simulink model "q_torsion"  (R2024a)
settings: Solver=ode1  StartTime=0.0  StopTime=5  FixedStep=0.002  RelTol=1e-3  EnableMultiTasking=on
values from neighbouring files (symbols this model uses):
  K = db2mag(12.15)    [pid_design.m]    (also in setup_torsion.m = d_torsion_1d_lqr(A,B))
  K_AMP = 1    [setup_torsion.m]
  K_ENC = 0    [config_srv02.m]
  VMAX_AMP = 0    [config_srv02.m]
  VMAX_DAC = 10    [setup_torsion.m]
  wcf = 2 * pi * 50.0    (= 314.159265359)    [setup_torsion.m]
  zetaf = 0.9    [setup_torsion.m]
undefined symbols (not defined in the file or in its folder): HIL, qc_get_step_size
libraries: quarc_library x9, simulink_extras x3
settings Model: SimulationMode=external  ExtModeTrigDuration=10000  Creator=MLevis  LastModifiedBy=quarc_user
settings SolverCC: AlgebraicLoopSolver=TrustRegion  PositivePriorityOrder=on
settings DataIOCC: LimitDataPoints=on  SaveFormat=Array  SignalLoggingSaveFormat=ModelDataLogs  ReturnWorkspaceOutputs=off
settings OptimizationCC: ExpressionDepthLimit=2147483647  InitFltsAndDblsToZero=on
settings DebuggingCC: SaveWithParameterizedLinksMsg=none  UnderspecifiedInitializationDetection=Classic  MergeDetectMultiDrivingBlocksExec=none  SolverPrmCheckMsg=warning  FcnCallInpInsideContextMsg=warning  UnconnectedInputMsg=warning  UnconnectedOutputMsg=warning  UnconnectedLineMsg=warning  StateNameClashWarn=warning  SFUnexpectedBacktrackingDiag=warning  SFNoUnconditionalDefaultTransitionDiag=warning  SFExecutionAtInitializationDiag=none  ArithmeticOperatorsInVariantConditions=warning
settings ModelReferenceCC: PropagateSignalLabelsOutOfModel=off
settings SFSimCC: SimUseLocalCustomCode=off  CustomCodeUndefinedFunction=UseInterfaceOnly
settings RTWCC: Description=QUARC Win64 Target Using Toolchain  SystemTargetFile=quarc_win64.tlc  TemplateMakefile=quarc_default_tmf  RTWUseLocalCustomCode=off  Toolchain=QUARC win64 | nmake (64-bit Windows)  BuildConfiguration=Faster Runs  GPUComputeCapability=3.5
settings CodeAppCC: StateflowObjectComments=on
settings STFCustomTargetCC: TargetLangStandard=C89/C90 (ANSI)  ConcurrentExecutionCompliant=on  SystemTargetFile=quarc_win64.tlc
settings GRTTargetCC: TargetLangStandard=C89/C90 (ANSI)  ParMdlRefBuildCompliant=off  CompOptLevelCompliant=off  CombineOutputUpdateFcns=off  MatFileLogging=off  CPPClassGenCompliant=off  GRTInterface=on  ExtMode=on  ExtModeMexFile=quarc_comm
settings ConfigComp: CovMetricSettings=dw  CovSaveCumulativeToWorkspaceVar=on  CovSaveSingleToWorkspaceVar=on  CovExternalEMLEnable=off

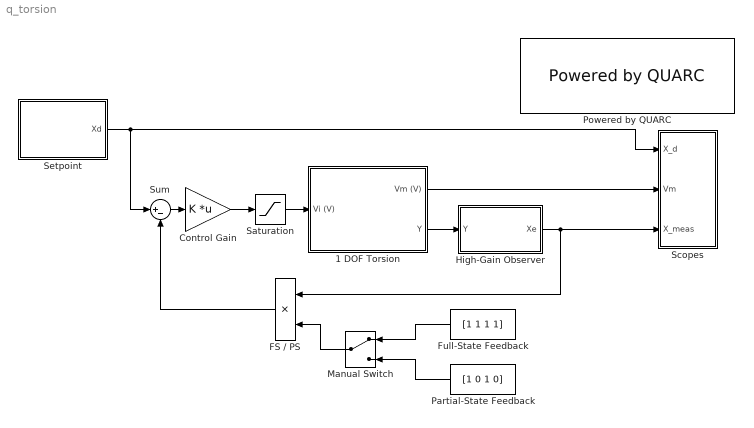
== system q_torsion ==
  1 DOF Torsion : Subsystem
  Control Gain : Gain  Gain=K  Multiplication=Matrix(K*u)  SaturateOnIntegerOverflow=on  OutDataTypeStr=Inherit: Same as input  ParamDataTypeStr=Inherit: Same as input
  FS / PS : Product  RndMeth=Zero
  Full-State Feedback : Constant  Value=[1 1 1 1]
  High-Gain Observer : Subsystem
  Manual Switch : ManualSwitch
  Partial-State Feedback : Constant  Value=[1 0 1 0]
  Powered by QUARC : quarc_library/Logos/Powered by QUARC
  Saturation : Saturate  UpperLimit=10  LowerLimit=-10
  Scopes : Subsystem
  Setpoint : Subsystem
  Sum : Sum  Inputs=|+-
  wires:
  1 DOF Torsion/2(Y) -> High-Gain Observer/1(Y)
  High-Gain Observer/1(Xe) -> Scopes/3(X_meas), FS / PS/1
  1 DOF Torsion/1(Vm (V)) -> Scopes/2(Vm)
  Setpoint/1(Xd) -> Scopes/1(X_d), Sum/1
  Full-State Feedback/1 -> Manual Switch/1
  Partial-State Feedback/1 -> Manual Switch/2
  Control Gain/1 -> Saturation/1
  Manual Switch/1 -> FS / PS/2
  FS / PS/1 -> Sum/2
  Sum/1 -> Control Gain/1
  Saturation/1 -> 1 DOF Torsion/1(Vi (V))

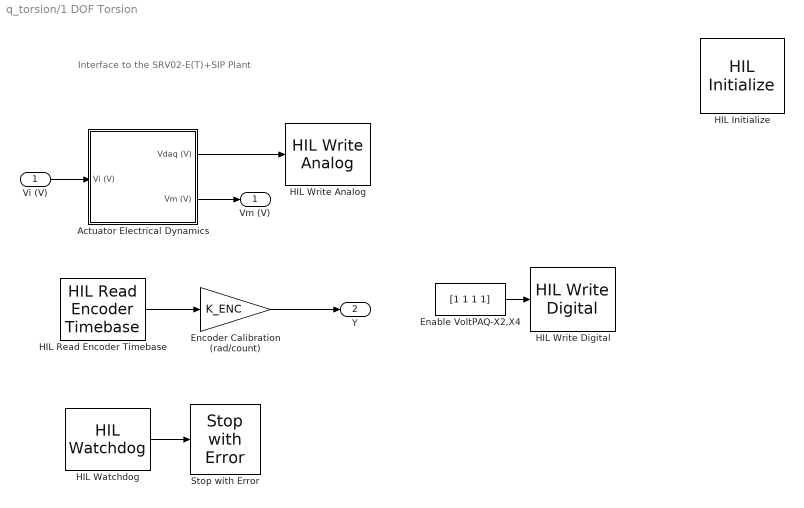
== system q_torsion/1 DOF Torsion ==
  note: Interface to the SRV02-E(T)+SIP Plant
  Vi (V) : Inport
  Actuator Electrical Dynamics : Subsystem
  Enable VoltPAQ-X2,X4 : Constant  Value=[1 1 1 1]
  Encoder Calibration (rad/count) : Gain  Gain=K_ENC  SaturateOnIntegerOverflow=on  OutDataTypeStr=Inherit: Same as input  ParamDataTypeStr=Inherit: Same as input
  HIL Initialize : quarc_library/Data Acquisition/Generic/Configuration/HIL Initialize  object_name=HIL-1  board_type=q2_usb  board_number=0  board_options=d0=digital;d1=digital;led=auto;update_rate=normal  exclusive=off  active=off  hardware_clocks=[0:2]  clock_modes=[]  initial_clock_frequencies=[]  set_clock_params_at_start=off  set_clock_params_at_switch_in=off  set_clock_frequencies_at_start=off  set_clock_frequencies_at_switch_in=off  analog_input_channels=[0:1]  analog_input_configurations=[]  analog_input_maximums=10  analog_input_minimums=-10  set_analog_input_params_at_start=on  set_analog_input_params_at_switch_in=off  analog_output_channels=[0:1]  analog_output_maximums=10  analog_output_minimums=-10  initial_analog_outputs=[0]  final_analog_outputs=[0]  watchdog_analog_outputs=0  set_analog_output_params_at_start=on  set_analog_output_params_at_switch_in=off  set_analog_outputs_at_start=on  set_analog_outputs_at_switch_in=off  set_analog_outputs_at_terminate=on  set_analog_outputs_at_switch_out=off  set_analog_outputs_on_watchdog=on  digital_input_channels=[]  digital_output_channels=[0:7]  digital_output_configuration=[]  initial_digital_outputs=[0]  final_digital_outputs=[0]  watchdog_digital_outputs=[0]  set_digital_output_params_at_start=off  set_digital_output_params_at_switch_in=off  set_digital_outputs_at_start=on  set_digital_outputs_at_switch_in=off  set_digital_outputs_at_terminate=on  set_digital_outputs_at_switch_out=off  set_digital_outputs_on_watchdog=on  encoder_channels=[0:1]  quadrature=[4]  encoder_filter_frequency=[]  initial_encoder_counts=[0]  set_encoder_params_at_start=on  set_encoder_params_at_switch_in=off  set_encoder_counts_at_start=on  set_encoder_counts_at_switch_in=off  pwm_channels=[]  pwm_modes=[0]  pwm_frequency=1/0.020  pwm_configuration=[]  pwm_alignment=[]  pwm_polarity=[]  pwm_leading_deadband=[]  pwm_trailing_deadband=[]  initial_pwm_outputs=[0]  final_pwm_outputs=[0]  watchdog_pwm_outputs=[0]  set_pwm_params_at_start=on  set_pwm_params_at_switch_in=off  set_pwm_outputs_at_start=on  set_pwm_outputs_at_switch_in=off  set_pwm_outputs_at_terminate=on  set_pwm_outputs_at_switch_out=off  set_pwm_outputs_on_watchdog=off  other_output_channels=[]  initial_other_outputs=[]  final_other_outputs=[]  watchdog_other_outputs=[]  set_other_outputs_at_start=off  set_other_outputs_at_switch_in=off  set_other_outputs_at_terminate=off  set_other_outputs_at_switch_out=off  set_other_outputs_on_watchdog=off
  HIL Read Encoder Timebase : quarc_library/Data Acquisition/Generic/Timebases/HIL Read Encoder Timebase  object_name=HIL-1  clock=0  channels=[0:1]  active=on  vector_output=on  data_type_mode=Inherit via back propagation  data_type=double  overflow_mode=Error on overflow  samples_in_buffer=max(ceil(1/qc_get_step_size), 1)
  HIL Watchdog : quarc_library/Data Acquisition/Generic/Watchdog/HIL Watchdog  object_name=HIL-1  timeout=10*qc_get_step_size  sample_time=qc_get_step_size  active=off
      settings: AttributesFormatString=(%<object_name>)  SourceProductName=QUARC Targets
  HIL Write Analog : quarc_library/Data Acquisition/Generic/Immediate I//O/HIL Write Analog  object_name=HIL-1  channels=0  sample_time=-1  active=off  vector_input=off
  HIL Write Digital : quarc_library/Data Acquisition/Generic/Immediate I//O/HIL Write Digital  object_name=HIL-1  channels=[0:3]  sample_time=-1  active=off  vector_input=on
      settings: SourceProductName=QUARC Targets
  Stop with Error : quarc_library/Sinks/Error Handling/Stop with Error  message_type=Fixed error message  message=Stopped by watchdog.
      settings: AttributesFormatString="\"%<message>\""  SourceProductName=QUARC Targets
  Vm (V) : Outport
  Y : Outport  Port=2
  wires:
  HIL Watchdog/1 -> Stop with Error/1
  Actuator Electrical Dynamics/1(Vdaq (V)) -> HIL Write Analog/1
  Actuator Electrical Dynamics/2(Vm (V)) -> Vm (V)/1
  HIL Read Encoder Timebase/1 -> Encoder Calibration (rad/count)/1
  Encoder Calibration (rad/count)/1 -> Y/1
  Enable VoltPAQ-X2,X4/1 -> HIL Write Digital/1
  Vi (V)/1 -> Actuator Electrical Dynamics/1(Vi (V))

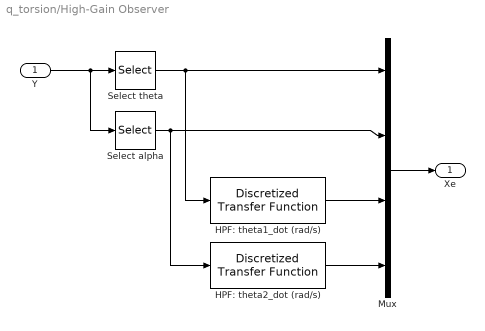
== system q_torsion/High-Gain Observer ==
  Y : Inport
  HPF: theta1_dot (rad/s) : quarc_library/Discrete/Discretized Transfer Function  num=[wcf^2 0]  den=[1 2*zetaf*wcf wcf^2]  method=tustin  Ts=qc_get_step_size
      settings: SourceProductName=QUARC Targets
  HPF: theta2_dot (rad/s) : quarc_library/Discrete/Discretized Transfer Function  num=[wcf^2 0]  den=[1 2*zetaf*wcf wcf^2]  method=tustin  Ts=qc_get_step_size
      settings: SourceProductName=QUARC Targets
  Mux : Mux
  Select alpha : Selector  InputPortWidth=2  IndexOptions=Index vector (dialog)  Indices=2  OutputSizes=1
  Select theta : Selector  InputPortWidth=2  IndexOptions=Index vector (dialog)  Indices=1  OutputSizes=1
  Xe : Outport
  wires:
  HPF: theta2_dot (rad/s)/1 -> Mux/4
  Select theta/1 -> Mux/1, HPF: theta1_dot (rad/s)/1
  HPF: theta1_dot (rad/s)/1 -> Mux/3
  Y/1 -> Select theta/1, Select alpha/1
  Mux/1 -> Xe/1
  Select alpha/1 -> HPF: theta2_dot (rad/s)/1, Mux/2

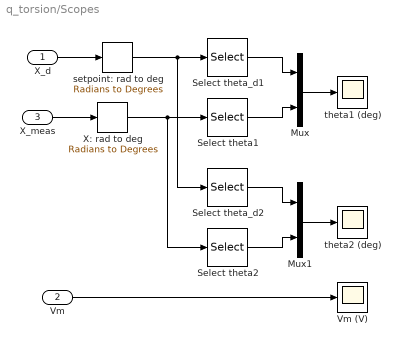
== system q_torsion/Scopes ==
  X_d : Inport
  Vm : Inport  Port=2
  X_meas : Inport  Port=3
  Mux : Mux  Inputs=2
  Mux1 : Mux  Inputs=2
  Select theta1 : Selector  InputPortWidth=4  IndexOptions=Index vector (dialog)  Indices=1  OutputSizes=1
  Select theta2 : Selector  InputPortWidth=4  IndexOptions=Index vector (dialog)  Indices=2  OutputSizes=1
  Select theta_d1 : Selector  InputPortWidth=4  IndexOptions=Index vector (dialog)  Indices=1  OutputSizes=1
  Select theta_d2 : Selector  InputPortWidth=4  IndexOptions=Index vector (dialog)  Indices=2  OutputSizes=1
  Vm (V) : Scope
  X: rad to deg : simulink_extras/Transformations/Radians to Degrees
  setpoint: rad to deg : simulink_extras/Transformations/Radians to Degrees
  theta1 (deg) : Scope
  theta2 (deg) : Scope
  wires:
  X_meas/1 -> X: rad to deg/1
  Mux/1 -> theta1 (deg)/1
  X_d/1 -> setpoint: rad to deg/1
  Vm/1 -> Vm (V)/1
  Mux1/1 -> theta2 (deg)/1
  setpoint: rad to deg/1 -> Select theta_d1/1, Select theta_d2/1
  Select theta_d1/1 -> Mux/1
  Select theta_d2/1 -> Mux1/1
  Select theta1/1 -> Mux/2
  Select theta2/1 -> Mux1/2
  X: rad to deg/1 -> Select theta1/1, Select theta2/1

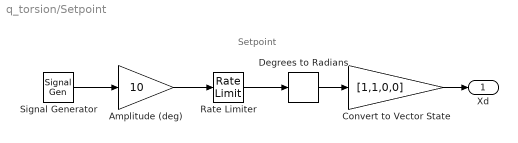
== system q_torsion/Setpoint ==
  note: Setpoint
  Amplitude (deg) : Gain  Gain=10  SaturateOnIntegerOverflow=on  OutDataTypeStr=Inherit: Same as input  ParamDataTypeStr=Inherit: Same as input
  Convert to Vector State : Gain  Gain=[1,1,0,0]
  Degrees to Radians : simulink_extras/Transformations/Degrees to Radians
  Rate Limiter : RateLimiter  RisingSlewLimit=5*180  FallingSlewLimit=-5*180  SampleTimeMode=inherited
  Signal Generator : SignalGenerator  WaveForm=square  Frequency=0.5
  Xd : Outport
  wires:
  Convert to Vector State/1 -> Xd/1
  Signal Generator/1 -> Amplitude (deg)/1
  Amplitude (deg)/1 -> Rate Limiter/1
  Rate Limiter/1 -> Degrees to Radians/1
  Degrees to Radians/1 -> Convert to Vector State/1

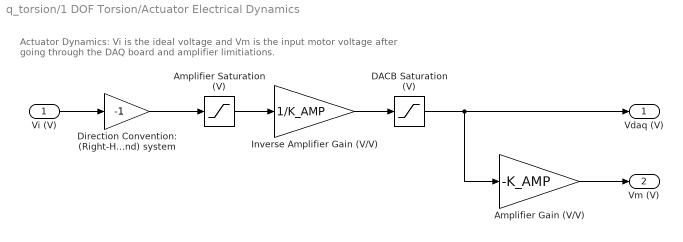
== system q_torsion/1 DOF Torsion/Actuator Electrical Dynamics ==
  note: Actuator Dynamics: Vi is the ideal voltage and Vm is the
      | input motor voltage after going through the DAQ board and amplifier limitiations.
  Vi (V) : Inport
  Amplifier Gain (V/V) : Gain  Gain=-K_AMP
  Amplifier Saturation (V) : Saturate  UpperLimit=VMAX_AMP  LowerLimit=-VMAX_AMP
  DACB Saturation (V) : Saturate  UpperLimit=VMAX_DAC  LowerLimit=-VMAX_DAC
  Direction Convention: (Right-Hand) system : Gain  Gain=-1  SaturateOnIntegerOverflow=on  OutDataTypeStr=Inherit: Same as input  ParamDataTypeStr=Inherit: Same as input
  Inverse Amplifier Gain (V/V) : Gain  Gain=1/K_AMP
  Vdaq (V) : Outport
  Vm (V) : Outport  Port=2
  wires:
  Direction Convention: (Right-Hand) system/1 -> Amplifier Saturation (V)/1
  Amplifier Gain (V/V)/1 -> Vm (V)/1
  DACB Saturation (V)/1 -> Vdaq (V)/1, Amplifier Gain (V/V)/1
  Inverse Amplifier Gain (V/V)/1 -> DACB Saturation (V)/1
  Vi (V)/1 -> Direction Convention: (Right-Hand) system/1
  Amplifier Saturation (V)/1 -> Inverse Amplifier Gain (V/V)/1
